simulink model "adc_to_10gbe"  (Simulink 7.4)
settings: Solver=ode45  StartTime=0.0  StopTime=200000  RelTol=1e-3
undefined symbols (not defined in the file): ROACH
libraries: xbsIndex_r4 x112, xps_library x77, casper_library_misc x6, xbsReplacements_r4 x3
(part 2 of 2)

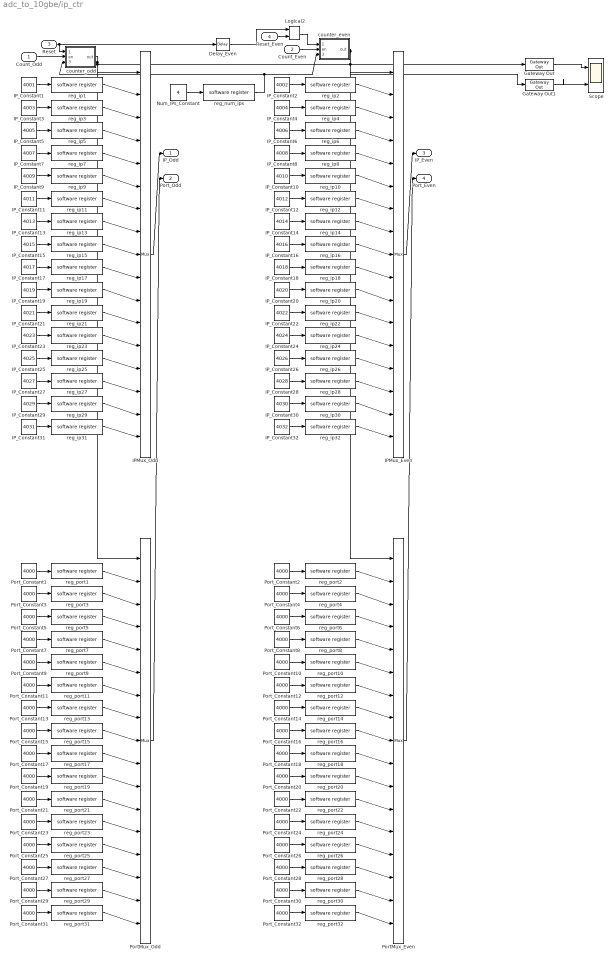
== system adc_to_10gbe/ip_ctr ==
  Count_Odd : Inport  OutDataType=sfix(16)  OutScaling=2^0
  Count_Even : Inport  Port=2  OutDataType=sfix(16)  OutScaling=2^0
  Reset : Inport  Port=3  OutDataType=sfix(16)  OutScaling=2^0
  Reset_Even : Inport  Port=4  OutDataType=sfix(16)  OutScaling=2^0
  Delay_Even : xbsIndex_r4/Delay  en=off  latency=4  dbl_ovrd=off  reg_retiming=off  block_type=delay
      settings: xl_area=[0, 0, 0, 0, 0, 0, 0]  block_version=10.1
  Gateway Out : xbsIndex_r4/Gateway Out  hdl_port=on  timing_constraint=None  locs_specified=off  LOCs={}  block_type=gatewayout
      settings: infoedit="Gateway out block.  Converts Xilinx fixed point inputs into ouputs of type Simulink integer, double, or fixed point.<P><P>Hardware notes:  In hardware these blocks become top level output ports or are discarded, depending on how they are configured."  xl_area=[0, 0, 0, 0, 0, 0, 0]  block_version=10.1
  Gateway Out1 : xbsIndex_r4/Gateway Out  hdl_port=on  timing_constraint=None  locs_specified=off  LOCs={}  block_type=gatewayout
      settings: infoedit="Gateway out block.  Converts Xilinx fixed point inputs into ouputs of type Simulink integer, double, or fixed point.<P><P>Hardware notes:  In hardware these blocks become top level output ports or are discarded, depending on how they are configured."  xl_area=[0, 0, 0, 0, 0, 0, 0]  block_version=10.1
  IPMux_Even : xbsIndex_r4/Mux  inputs=16  en=off  latency=3  precision=Full  arith_type="Signed  (2's comp)"  n_bits=8  bin_pt=2  quantization=Truncate  overflow=Wrap  dbl_ovrd=off  block_type=mux
      settings: xl_area=[0, 0, 0, 0, 0, 0, 0]  block_version=10.1
  IPMux_Odd : xbsIndex_r4/Mux  inputs=16  en=off  latency=3  precision=Full  arith_type="Signed  (2's comp)"  n_bits=8  bin_pt=2  quantization=Truncate  overflow=Wrap  dbl_ovrd=off  block_type=mux
      settings: xl_area=[0, 0, 0, 0, 0, 0, 0]  block_version=10.1
  IP_Constant1 : Constant  Value=4001  OutDataType=sfix(16)  OutScaling=2^0
  IP_Constant10 : Constant  Value=4010  OutDataType=sfix(16)  OutScaling=2^0
  IP_Constant11 : Constant  Value=4011  OutDataType=sfix(16)  OutScaling=2^0
  IP_Constant12 : Constant  Value=4012  OutDataType=sfix(16)  OutScaling=2^0
  IP_Constant13 : Constant  Value=4013  OutDataType=sfix(16)  OutScaling=2^0
  IP_Constant14 : Constant  Value=4014  OutDataType=sfix(16)  OutScaling=2^0
  IP_Constant15 : Constant  Value=4015  OutDataType=sfix(16)  OutScaling=2^0
  IP_Constant16 : Constant  Value=4016  OutDataType=sfix(16)  OutScaling=2^0
  IP_Constant17 : Constant  Value=4017  OutDataType=sfix(16)  OutScaling=2^0
  IP_Constant18 : Constant  Value=4018  OutDataType=sfix(16)  OutScaling=2^0
  IP_Constant19 : Constant  Value=4019  OutDataType=sfix(16)  OutScaling=2^0
  IP_Constant2 : Constant  Value=4002  OutDataType=sfix(16)  OutScaling=2^0
  IP_Constant20 : Constant  Value=4020  OutDataType=sfix(16)  OutScaling=2^0
  IP_Constant21 : Constant  Value=4021  OutDataType=sfix(16)  OutScaling=2^0
  IP_Constant22 : Constant  Value=4022  OutDataType=sfix(16)  OutScaling=2^0
  IP_Constant23 : Constant  Value=4023  OutDataType=sfix(16)  OutScaling=2^0
  IP_Constant24 : Constant  Value=4024  OutDataType=sfix(16)  OutScaling=2^0
  IP_Constant25 : Constant  Value=4025  OutDataType=sfix(16)  OutScaling=2^0
  IP_Constant26 : Constant  Value=4026  OutDataType=sfix(16)  OutScaling=2^0
  IP_Constant27 : Constant  Value=4027  OutDataType=sfix(16)  OutScaling=2^0
  IP_Constant28 : Constant  Value=4028  OutDataType=sfix(16)  OutScaling=2^0
  IP_Constant29 : Constant  Value=4029  OutDataType=sfix(16)  OutScaling=2^0
  IP_Constant3 : Constant  Value=4003  OutDataType=sfix(16)  OutScaling=2^0
  IP_Constant30 : Constant  Value=4030  OutDataType=sfix(16)  OutScaling=2^0
  IP_Constant31 : Constant  Value=4031  OutDataType=sfix(16)  OutScaling=2^0
  IP_Constant32 : Constant  Value=4032  OutDataType=sfix(16)  OutScaling=2^0
  IP_Constant4 : Constant  Value=4004  OutDataType=sfix(16)  OutScaling=2^0
  IP_Constant5 : Constant  Value=4005  OutDataType=sfix(16)  OutScaling=2^0
  IP_Constant6 : Constant  Value=4006  OutDataType=sfix(16)  OutScaling=2^0
  IP_Constant7 : Constant  Value=4007  OutDataType=sfix(16)  OutScaling=2^0
  IP_Constant8 : Constant  Value=4008  OutDataType=sfix(16)  OutScaling=2^0
  IP_Constant9 : Constant  Value=4009  OutDataType=sfix(16)  OutScaling=2^0
  Logical2 : xbsIndex_r4/Logical  logical_function=OR  inputs=2  en=off  latency=0  precision=Full  arith_type=Unsigned  n_bits=8  bin_pt=2  align_bp=on  dbl_ovrd=off  block_type=logical
      settings: xl_area=[0, 0, 0, 0, 0, 0, 0]  block_version=10.1
  Num_IPs_Constant : Constant  Value=4  OutDataType=sfix(16)  OutScaling=2^0
  PortMux_Even : xbsIndex_r4/Mux  inputs=16  en=off  latency=3  precision=Full  arith_type="Signed  (2's comp)"  n_bits=8  bin_pt=2  quantization=Truncate  overflow=Wrap  dbl_ovrd=off  block_type=mux
      settings: xl_area=[0, 0, 0, 0, 0, 0, 0]  block_version=10.1
  PortMux_Odd : xbsIndex_r4/Mux  inputs=16  en=off  latency=3  precision=Full  arith_type="Signed  (2's comp)"  n_bits=8  bin_pt=2  quantization=Truncate  overflow=Wrap  dbl_ovrd=off  block_type=mux
      settings: xl_area=[0, 0, 0, 0, 0, 0, 0]  block_version=10.1
  Port_Constant{1..32} (32 alike) : Constant  Value=4000  OutDataType=sfix(16)  OutScaling=2^0
  Scope : Scope  NumInputPorts=2
      settings: YMin=-5~-5  YMax=5~5  SaveName=ScopeData4
  counter_even : Subsystem
  counter_odd : Subsystem
  reg_ip1 : xps_library/software register  Tag=xps:sw_reg  SystemSampleTime=-1  io_dir=From Processor  arith_type=Unsigned  bitwidth=32  bin_pt=0  sample_period=1  gw_name=adc_to_10gbe_ip_ctr_reg_ip1_user_data_out
      link override adc_to_10gbe_ip_ctr_reg_ip1_user_data_out: arith_type=Unsigned  n_bits=32  bin_pt=0  period=1
      link override adc_to_10gbe_mod_ip_ctr_reg_ip1_user_data_out: arith_type=Unsigned  n_bits=32  bin_pt=0  period=1
  reg_ip10 : xps_library/software register  Tag=xps:sw_reg  SystemSampleTime=-1  io_dir=From Processor  arith_type=Unsigned  bitwidth=32  bin_pt=0  sample_period=1  gw_name=adc_to_10gbe_ip_ctr_reg_ip10_user_data_out
      link override adc_to_10gbe_ip_ctr_reg_ip10_user_data_out: arith_type=Unsigned  n_bits=32  bin_pt=0  period=1
      link override adc_to_10gbe_mod_ip_ctr_reg_ip10_user_data_out: arith_type=Unsigned  n_bits=32  bin_pt=0  period=1
  reg_ip11 : xps_library/software register  Tag=xps:sw_reg  SystemSampleTime=-1  io_dir=From Processor  arith_type=Unsigned  bitwidth=32  bin_pt=0  sample_period=1  gw_name=adc_to_10gbe_ip_ctr_reg_ip11_user_data_out
      link override adc_to_10gbe_ip_ctr_reg_ip11_user_data_out: arith_type=Unsigned  n_bits=32  bin_pt=0  period=1
      link override adc_to_10gbe_mod_ip_ctr_reg_ip11_user_data_out: arith_type=Unsigned  n_bits=32  bin_pt=0  period=1
  reg_ip12 : xps_library/software register  Tag=xps:sw_reg  SystemSampleTime=-1  io_dir=From Processor  arith_type=Unsigned  bitwidth=32  bin_pt=0  sample_period=1  gw_name=adc_to_10gbe_ip_ctr_reg_ip12_user_data_out
      link override adc_to_10gbe_ip_ctr_reg_ip12_user_data_out: arith_type=Unsigned  n_bits=32  bin_pt=0  period=1
      link override adc_to_10gbe_mod_ip_ctr_reg_ip12_user_data_out: arith_type=Unsigned  n_bits=32  bin_pt=0  period=1
  reg_ip13 : xps_library/software register  Tag=xps:sw_reg  SystemSampleTime=-1  io_dir=From Processor  arith_type=Unsigned  bitwidth=32  bin_pt=0  sample_period=1  gw_name=adc_to_10gbe_ip_ctr_reg_ip13_user_data_out
      link override adc_to_10gbe_ip_ctr_reg_ip13_user_data_out: arith_type=Unsigned  n_bits=32  bin_pt=0  period=1
      link override adc_to_10gbe_mod_ip_ctr_reg_ip13_user_data_out: arith_type=Unsigned  n_bits=32  bin_pt=0  period=1
  reg_ip14 : xps_library/software register  Tag=xps:sw_reg  SystemSampleTime=-1  io_dir=From Processor  arith_type=Unsigned  bitwidth=32  bin_pt=0  sample_period=1  gw_name=adc_to_10gbe_ip_ctr_reg_ip14_user_data_out
      link override adc_to_10gbe_ip_ctr_reg_ip14_user_data_out: arith_type=Unsigned  n_bits=32  bin_pt=0  period=1
      link override adc_to_10gbe_mod_ip_ctr_reg_ip14_user_data_out: arith_type=Unsigned  n_bits=32  bin_pt=0  period=1
  reg_ip15 : xps_library/software register  Tag=xps:sw_reg  SystemSampleTime=-1  io_dir=From Processor  arith_type=Unsigned  bitwidth=32  bin_pt=0  sample_period=1  gw_name=adc_to_10gbe_ip_ctr_reg_ip15_user_data_out
      link override adc_to_10gbe_ip_ctr_reg_ip15_user_data_out: arith_type=Unsigned  n_bits=32  bin_pt=0  period=1
      link override adc_to_10gbe_mod_ip_ctr_reg_ip15_user_data_out: arith_type=Unsigned  n_bits=32  bin_pt=0  period=1
  reg_ip16 : xps_library/software register  Tag=xps:sw_reg  SystemSampleTime=-1  io_dir=From Processor  arith_type=Unsigned  bitwidth=32  bin_pt=0  sample_period=1  gw_name=adc_to_10gbe_ip_ctr_reg_ip16_user_data_out
      link override adc_to_10gbe_ip_ctr_reg_ip16_user_data_out: arith_type=Unsigned  n_bits=32  bin_pt=0  period=1
      link override adc_to_10gbe_mod_ip_ctr_reg_ip16_user_data_out: arith_type=Unsigned  n_bits=32  bin_pt=0  period=1
  reg_ip17 : xps_library/software register  Tag=xps:sw_reg  SystemSampleTime=-1  io_dir=From Processor  arith_type=Unsigned  bitwidth=32  bin_pt=0  sample_period=1  gw_name=adc_to_10gbe_ip_ctr_reg_ip17_user_data_out
      link override adc_to_10gbe_ip_ctr_reg_ip17_user_data_out: arith_type=Unsigned  n_bits=32  bin_pt=0  period=1
      link override adc_to_10gbe_mod_ip_ctr_reg_ip17_user_data_out: arith_type=Unsigned  n_bits=32  bin_pt=0  period=1
  reg_ip18 : xps_library/software register  Tag=xps:sw_reg  SystemSampleTime=-1  io_dir=From Processor  arith_type=Unsigned  bitwidth=32  bin_pt=0  sample_period=1  gw_name=adc_to_10gbe_ip_ctr_reg_ip18_user_data_out
      link override adc_to_10gbe_ip_ctr_reg_ip18_user_data_out: arith_type=Unsigned  n_bits=32  bin_pt=0  period=1
      link override adc_to_10gbe_mod_ip_ctr_reg_ip18_user_data_out: arith_type=Unsigned  n_bits=32  bin_pt=0  period=1
  reg_ip19 : xps_library/software register  Tag=xps:sw_reg  SystemSampleTime=-1  io_dir=From Processor  arith_type=Unsigned  bitwidth=32  bin_pt=0  sample_period=1  gw_name=adc_to_10gbe_ip_ctr_reg_ip19_user_data_out
      link override adc_to_10gbe_ip_ctr_reg_ip19_user_data_out: arith_type=Unsigned  n_bits=32  bin_pt=0  period=1
      link override adc_to_10gbe_mod_ip_ctr_reg_ip19_user_data_out: arith_type=Unsigned  n_bits=32  bin_pt=0  period=1
  reg_ip2 : xps_library/software register  Tag=xps:sw_reg  SystemSampleTime=-1  io_dir=From Processor  arith_type=Unsigned  bitwidth=32  bin_pt=0  sample_period=1  gw_name=adc_to_10gbe_ip_ctr_reg_ip2_user_data_out
      link override adc_to_10gbe_ip_ctr_reg_ip2_user_data_out: arith_type=Unsigned  n_bits=32  bin_pt=0  period=1
      link override adc_to_10gbe_mod_ip_ctr_reg_ip2_user_data_out: arith_type=Unsigned  n_bits=32  bin_pt=0  period=1
  reg_ip20 : xps_library/software register  Tag=xps:sw_reg  SystemSampleTime=-1  io_dir=From Processor  arith_type=Unsigned  bitwidth=32  bin_pt=0  sample_period=1  gw_name=adc_to_10gbe_ip_ctr_reg_ip20_user_data_out
      link override adc_to_10gbe_ip_ctr_reg_ip20_user_data_out: arith_type=Unsigned  n_bits=32  bin_pt=0  period=1
      link override adc_to_10gbe_mod_ip_ctr_reg_ip20_user_data_out: arith_type=Unsigned  n_bits=32  bin_pt=0  period=1
  reg_ip21 : xps_library/software register  Tag=xps:sw_reg  SystemSampleTime=-1  io_dir=From Processor  arith_type=Unsigned  bitwidth=32  bin_pt=0  sample_period=1  gw_name=adc_to_10gbe_ip_ctr_reg_ip21_user_data_out
      link override adc_to_10gbe_ip_ctr_reg_ip21_user_data_out: arith_type=Unsigned  n_bits=32  bin_pt=0  period=1
      link override adc_to_10gbe_mod_ip_ctr_reg_ip21_user_data_out: arith_type=Unsigned  n_bits=32  bin_pt=0  period=1
  reg_ip22 : xps_library/software register  Tag=xps:sw_reg  SystemSampleTime=-1  io_dir=From Processor  arith_type=Unsigned  bitwidth=32  bin_pt=0  sample_period=1  gw_name=adc_to_10gbe_ip_ctr_reg_ip22_user_data_out
      link override adc_to_10gbe_ip_ctr_reg_ip22_user_data_out: arith_type=Unsigned  n_bits=32  bin_pt=0  period=1
      link override adc_to_10gbe_mod_ip_ctr_reg_ip22_user_data_out: arith_type=Unsigned  n_bits=32  bin_pt=0  period=1
  reg_ip23 : xps_library/software register  Tag=xps:sw_reg  SystemSampleTime=-1  io_dir=From Processor  arith_type=Unsigned  bitwidth=32  bin_pt=0  sample_period=1  gw_name=adc_to_10gbe_ip_ctr_reg_ip23_user_data_out
      link override adc_to_10gbe_ip_ctr_reg_ip23_user_data_out: arith_type=Unsigned  n_bits=32  bin_pt=0  period=1
      link override adc_to_10gbe_mod_ip_ctr_reg_ip23_user_data_out: arith_type=Unsigned  n_bits=32  bin_pt=0  period=1
  reg_ip24 : xps_library/software register  Tag=xps:sw_reg  SystemSampleTime=-1  io_dir=From Processor  arith_type=Unsigned  bitwidth=32  bin_pt=0  sample_period=1  gw_name=adc_to_10gbe_ip_ctr_reg_ip24_user_data_out
      link override adc_to_10gbe_ip_ctr_reg_ip24_user_data_out: arith_type=Unsigned  n_bits=32  bin_pt=0  period=1
      link override adc_to_10gbe_mod_ip_ctr_reg_ip24_user_data_out: arith_type=Unsigned  n_bits=32  bin_pt=0  period=1
  reg_ip25 : xps_library/software register  Tag=xps:sw_reg  SystemSampleTime=-1  io_dir=From Processor  arith_type=Unsigned  bitwidth=32  bin_pt=0  sample_period=1  gw_name=adc_to_10gbe_ip_ctr_reg_ip25_user_data_out
      link override adc_to_10gbe_ip_ctr_reg_ip25_user_data_out: arith_type=Unsigned  n_bits=32  bin_pt=0  period=1
      link override adc_to_10gbe_mod_ip_ctr_reg_ip25_user_data_out: arith_type=Unsigned  n_bits=32  bin_pt=0  period=1
  reg_ip26 : xps_library/software register  Tag=xps:sw_reg  SystemSampleTime=-1  io_dir=From Processor  arith_type=Unsigned  bitwidth=32  bin_pt=0  sample_period=1  gw_name=adc_to_10gbe_ip_ctr_reg_ip26_user_data_out
      link override adc_to_10gbe_ip_ctr_reg_ip26_user_data_out: arith_type=Unsigned  n_bits=32  bin_pt=0  period=1
      link override adc_to_10gbe_mod_ip_ctr_reg_ip26_user_data_out: arith_type=Unsigned  n_bits=32  bin_pt=0  period=1
  reg_ip27 : xps_library/software register  Tag=xps:sw_reg  SystemSampleTime=-1  io_dir=From Processor  arith_type=Unsigned  bitwidth=32  bin_pt=0  sample_period=1  gw_name=adc_to_10gbe_ip_ctr_reg_ip27_user_data_out
      link override adc_to_10gbe_ip_ctr_reg_ip27_user_data_out: arith_type=Unsigned  n_bits=32  bin_pt=0  period=1
      link override adc_to_10gbe_mod_ip_ctr_reg_ip27_user_data_out: arith_type=Unsigned  n_bits=32  bin_pt=0  period=1
  reg_ip28 : xps_library/software register  Tag=xps:sw_reg  SystemSampleTime=-1  io_dir=From Processor  arith_type=Unsigned  bitwidth=32  bin_pt=0  sample_period=1  gw_name=adc_to_10gbe_ip_ctr_reg_ip28_user_data_out
      link override adc_to_10gbe_ip_ctr_reg_ip28_user_data_out: arith_type=Unsigned  n_bits=32  bin_pt=0  period=1
      link override adc_to_10gbe_mod_ip_ctr_reg_ip28_user_data_out: arith_type=Unsigned  n_bits=32  bin_pt=0  period=1
  reg_ip29 : xps_library/software register  Tag=xps:sw_reg  SystemSampleTime=-1  io_dir=From Processor  arith_type=Unsigned  bitwidth=32  bin_pt=0  sample_period=1  gw_name=adc_to_10gbe_ip_ctr_reg_ip29_user_data_out
      link override adc_to_10gbe_ip_ctr_reg_ip29_user_data_out: arith_type=Unsigned  n_bits=32  bin_pt=0  period=1
      link override adc_to_10gbe_mod_ip_ctr_reg_ip29_user_data_out: arith_type=Unsigned  n_bits=32  bin_pt=0  period=1
  reg_ip3 : xps_library/software register  Tag=xps:sw_reg  SystemSampleTime=-1  io_dir=From Processor  arith_type=Unsigned  bitwidth=32  bin_pt=0  sample_period=1  gw_name=adc_to_10gbe_ip_ctr_reg_ip3_user_data_out
      link override adc_to_10gbe_ip_ctr_reg_ip3_user_data_out: arith_type=Unsigned  n_bits=32  bin_pt=0  period=1
      link override adc_to_10gbe_mod_ip_ctr_reg_ip3_user_data_out: arith_type=Unsigned  n_bits=32  bin_pt=0  period=1
  reg_ip30 : xps_library/software register  Tag=xps:sw_reg  SystemSampleTime=-1  io_dir=From Processor  arith_type=Unsigned  bitwidth=32  bin_pt=0  sample_period=1  gw_name=adc_to_10gbe_ip_ctr_reg_ip30_user_data_out
      link override adc_to_10gbe_ip_ctr_reg_ip30_user_data_out: arith_type=Unsigned  n_bits=32  bin_pt=0  period=1
      link override adc_to_10gbe_mod_ip_ctr_reg_ip30_user_data_out: arith_type=Unsigned  n_bits=32  bin_pt=0  period=1
  reg_ip31 : xps_library/software register  Tag=xps:sw_reg  SystemSampleTime=-1  io_dir=From Processor  arith_type=Unsigned  bitwidth=32  bin_pt=0  sample_period=1  gw_name=adc_to_10gbe_ip_ctr_reg_ip31_user_data_out
      link override adc_to_10gbe_ip_ctr_reg_ip31_user_data_out: arith_type=Unsigned  n_bits=32  bin_pt=0  period=1
      link override adc_to_10gbe_mod_ip_ctr_reg_ip31_user_data_out: arith_type=Unsigned  n_bits=32  bin_pt=0  period=1
  reg_ip32 : xps_library/software register  Tag=xps:sw_reg  SystemSampleTime=-1  io_dir=From Processor  arith_type=Unsigned  bitwidth=32  bin_pt=0  sample_period=1  gw_name=adc_to_10gbe_ip_ctr_reg_ip32_user_data_out
      link override adc_to_10gbe_ip_ctr_reg_ip32_user_data_out: arith_type=Unsigned  n_bits=32  bin_pt=0  period=1
      link override adc_to_10gbe_mod_ip_ctr_reg_ip32_user_data_out: arith_type=Unsigned  n_bits=32  bin_pt=0  period=1
  reg_ip4 : xps_library/software register  Tag=xps:sw_reg  SystemSampleTime=-1  io_dir=From Processor  arith_type=Unsigned  bitwidth=32  bin_pt=0  sample_period=1  gw_name=adc_to_10gbe_ip_ctr_reg_ip4_user_data_out
      link override adc_to_10gbe_ip_ctr_reg_ip4_user_data_out: arith_type=Unsigned  n_bits=32  bin_pt=0  period=1
      link override adc_to_10gbe_mod_ip_ctr_reg_ip4_user_data_out: arith_type=Unsigned  n_bits=32  bin_pt=0  period=1
  reg_ip5 : xps_library/software register  Tag=xps:sw_reg  SystemSampleTime=-1  io_dir=From Processor  arith_type=Unsigned  bitwidth=32  bin_pt=0  sample_period=1  gw_name=adc_to_10gbe_ip_ctr_reg_ip5_user_data_out
      link override adc_to_10gbe_ip_ctr_reg_ip5_user_data_out: arith_type=Unsigned  n_bits=32  bin_pt=0  period=1
      link override adc_to_10gbe_mod_ip_ctr_reg_ip5_user_data_out: arith_type=Unsigned  n_bits=32  bin_pt=0  period=1
  reg_ip6 : xps_library/software register  Tag=xps:sw_reg  SystemSampleTime=-1  io_dir=From Processor  arith_type=Unsigned  bitwidth=32  bin_pt=0  sample_period=1  gw_name=adc_to_10gbe_ip_ctr_reg_ip6_user_data_out
      link override adc_to_10gbe_ip_ctr_reg_ip6_user_data_out: arith_type=Unsigned  n_bits=32  bin_pt=0  period=1
      link override adc_to_10gbe_mod_ip_ctr_reg_ip6_user_data_out: arith_type=Unsigned  n_bits=32  bin_pt=0  period=1
  reg_ip7 : xps_library/software register  Tag=xps:sw_reg  SystemSampleTime=-1  io_dir=From Processor  arith_type=Unsigned  bitwidth=32  bin_pt=0  sample_period=1  gw_name=adc_to_10gbe_ip_ctr_reg_ip7_user_data_out
      link override adc_to_10gbe_ip_ctr_reg_ip7_user_data_out: arith_type=Unsigned  n_bits=32  bin_pt=0  period=1
      link override adc_to_10gbe_mod_ip_ctr_reg_ip7_user_data_out: arith_type=Unsigned  n_bits=32  bin_pt=0  period=1
  reg_ip8 : xps_library/software register  Tag=xps:sw_reg  SystemSampleTime=-1  io_dir=From Processor  arith_type=Unsigned  bitwidth=32  bin_pt=0  sample_period=1  gw_name=adc_to_10gbe_ip_ctr_reg_ip8_user_data_out
      link override adc_to_10gbe_ip_ctr_reg_ip8_user_data_out: arith_type=Unsigned  n_bits=32  bin_pt=0  period=1
      link override adc_to_10gbe_mod_ip_ctr_reg_ip8_user_data_out: arith_type=Unsigned  n_bits=32  bin_pt=0  period=1
  reg_ip9 : xps_library/software register  Tag=xps:sw_reg  SystemSampleTime=-1  io_dir=From Processor  arith_type=Unsigned  bitwidth=32  bin_pt=0  sample_period=1  gw_name=adc_to_10gbe_ip_ctr_reg_ip9_user_data_out
      link override adc_to_10gbe_ip_ctr_reg_ip9_user_data_out: arith_type=Unsigned  n_bits=32  bin_pt=0  period=1
      link override adc_to_10gbe_mod_ip_ctr_reg_ip9_user_data_out: arith_type=Unsigned  n_bits=32  bin_pt=0  period=1
  reg_num_ips : xps_library/software register  Tag=xps:sw_reg  SystemSampleTime=-1  io_dir=From Processor  arith_type=Unsigned  bitwidth=32  bin_pt=0  sample_period=1  gw_name=adc_to_10gbe_ip_ctr_reg_num_ips_user_data_out
      link override adc_to_10gbe_ip_ctr_reg_num_ips_user_data_out: arith_type=Unsigned  n_bits=32  bin_pt=0  period=1
      link override adc_to_10gbe_mod_ip_ctr_reg_num_ips_user_data_out: arith_type=Unsigned  n_bits=32  bin_pt=0  period=1
  reg_port1 : xps_library/software register  Tag=xps:sw_reg  SystemSampleTime=-1  io_dir=From Processor  arith_type=Unsigned  bitwidth=32  bin_pt=0  sample_period=1  gw_name=adc_to_10gbe_ip_ctr_reg_port1_user_data_out
      link override adc_to_10gbe_ip_ctr_reg_port1_user_data_out: arith_type=Unsigned  n_bits=32  bin_pt=0  period=1
      link override adc_to_10gbe_mod_ip_ctr_reg_port1_user_data_out: arith_type=Unsigned  n_bits=32  bin_pt=0  period=1
  reg_port10 : xps_library/software register  Tag=xps:sw_reg  SystemSampleTime=-1  io_dir=From Processor  arith_type=Unsigned  bitwidth=32  bin_pt=0  sample_period=1  gw_name=adc_to_10gbe_ip_ctr_reg_port10_user_data_out
      link override adc_to_10gbe_ip_ctr_reg_port10_user_data_out: arith_type=Unsigned  n_bits=32  bin_pt=0  period=1
      link override adc_to_10gbe_mod_ip_ctr_reg_port10_user_data_out: arith_type=Unsigned  n_bits=32  bin_pt=0  period=1
  reg_port11 : xps_library/software register  Tag=xps:sw_reg  SystemSampleTime=-1  io_dir=From Processor  arith_type=Unsigned  bitwidth=32  bin_pt=0  sample_period=1  gw_name=adc_to_10gbe_ip_ctr_reg_port11_user_data_out
      link override adc_to_10gbe_ip_ctr_reg_port11_user_data_out: arith_type=Unsigned  n_bits=32  bin_pt=0  period=1
      link override adc_to_10gbe_mod_ip_ctr_reg_port11_user_data_out: arith_type=Unsigned  n_bits=32  bin_pt=0  period=1
  reg_port12 : xps_library/software register  Tag=xps:sw_reg  SystemSampleTime=-1  io_dir=From Processor  arith_type=Unsigned  bitwidth=32  bin_pt=0  sample_period=1  gw_name=adc_to_10gbe_ip_ctr_reg_port12_user_data_out
      link override adc_to_10gbe_ip_ctr_reg_port12_user_data_out: arith_type=Unsigned  n_bits=32  bin_pt=0  period=1
      link override adc_to_10gbe_mod_ip_ctr_reg_port12_user_data_out: arith_type=Unsigned  n_bits=32  bin_pt=0  period=1
  reg_port13 : xps_library/software register  Tag=xps:sw_reg  SystemSampleTime=-1  io_dir=From Processor  arith_type=Unsigned  bitwidth=32  bin_pt=0  sample_period=1  gw_name=adc_to_10gbe_ip_ctr_reg_port13_user_data_out
      link override adc_to_10gbe_ip_ctr_reg_port13_user_data_out: arith_type=Unsigned  n_bits=32  bin_pt=0  period=1
      link override adc_to_10gbe_mod_ip_ctr_reg_port13_user_data_out: arith_type=Unsigned  n_bits=32  bin_pt=0  period=1
  reg_port14 : xps_library/software register  Tag=xps:sw_reg  SystemSampleTime=-1  io_dir=From Processor  arith_type=Unsigned  bitwidth=32  bin_pt=0  sample_period=1  gw_name=adc_to_10gbe_ip_ctr_reg_port14_user_data_out
      link override adc_to_10gbe_ip_ctr_reg_port14_user_data_out: arith_type=Unsigned  n_bits=32  bin_pt=0  period=1
      link override adc_to_10gbe_mod_ip_ctr_reg_port14_user_data_out: arith_type=Unsigned  n_bits=32  bin_pt=0  period=1
  reg_port15 : xps_library/software register  Tag=xps:sw_reg  SystemSampleTime=-1  io_dir=From Processor  arith_type=Unsigned  bitwidth=32  bin_pt=0  sample_period=1  gw_name=adc_to_10gbe_ip_ctr_reg_port15_user_data_out
      link override adc_to_10gbe_ip_ctr_reg_port15_user_data_out: arith_type=Unsigned  n_bits=32  bin_pt=0  period=1
      link override adc_to_10gbe_mod_ip_ctr_reg_port15_user_data_out: arith_type=Unsigned  n_bits=32  bin_pt=0  period=1
  reg_port16 : xps_library/software register  Tag=xps:sw_reg  SystemSampleTime=-1  io_dir=From Processor  arith_type=Unsigned  bitwidth=32  bin_pt=0  sample_period=1  gw_name=adc_to_10gbe_ip_ctr_reg_port16_user_data_out
      link override adc_to_10gbe_ip_ctr_reg_port16_user_data_out: arith_type=Unsigned  n_bits=32  bin_pt=0  period=1
      link override adc_to_10gbe_mod_ip_ctr_reg_port16_user_data_out: arith_type=Unsigned  n_bits=32  bin_pt=0  period=1
  reg_port17 : xps_library/software register  Tag=xps:sw_reg  SystemSampleTime=-1  io_dir=From Processor  arith_type=Unsigned  bitwidth=32  bin_pt=0  sample_period=1  gw_name=adc_to_10gbe_ip_ctr_reg_port17_user_data_out
      link override adc_to_10gbe_ip_ctr_reg_port17_user_data_out: arith_type=Unsigned  n_bits=32  bin_pt=0  period=1
      link override adc_to_10gbe_mod_ip_ctr_reg_port17_user_data_out: arith_type=Unsigned  n_bits=32  bin_pt=0  period=1
  reg_port18 : xps_library/software register  Tag=xps:sw_reg  SystemSampleTime=-1  io_dir=From Processor  arith_type=Unsigned  bitwidth=32  bin_pt=0  sample_period=1  gw_name=adc_to_10gbe_ip_ctr_reg_port18_user_data_out
      link override adc_to_10gbe_ip_ctr_reg_port18_user_data_out: arith_type=Unsigned  n_bits=32  bin_pt=0  period=1
      link override adc_to_10gbe_mod_ip_ctr_reg_port18_user_data_out: arith_type=Unsigned  n_bits=32  bin_pt=0  period=1
  reg_port19 : xps_library/software register  Tag=xps:sw_reg  SystemSampleTime=-1  io_dir=From Processor  arith_type=Unsigned  bitwidth=32  bin_pt=0  sample_period=1  gw_name=adc_to_10gbe_ip_ctr_reg_port19_user_data_out
      link override adc_to_10gbe_ip_ctr_reg_port19_user_data_out: arith_type=Unsigned  n_bits=32  bin_pt=0  period=1
      link override adc_to_10gbe_mod_ip_ctr_reg_port19_user_data_out: arith_type=Unsigned  n_bits=32  bin_pt=0  period=1
  reg_port2 : xps_library/software register  Tag=xps:sw_reg  SystemSampleTime=-1  io_dir=From Processor  arith_type=Unsigned  bitwidth=32  bin_pt=0  sample_period=1  gw_name=adc_to_10gbe_ip_ctr_reg_port2_user_data_out
      link override adc_to_10gbe_ip_ctr_reg_port2_user_data_out: arith_type=Unsigned  n_bits=32  bin_pt=0  period=1
      link override adc_to_10gbe_mod_ip_ctr_reg_port2_user_data_out: arith_type=Unsigned  n_bits=32  bin_pt=0  period=1
  reg_port20 : xps_library/software register  Tag=xps:sw_reg  SystemSampleTime=-1  io_dir=From Processor  arith_type=Unsigned  bitwidth=32  bin_pt=0  sample_period=1  gw_name=adc_to_10gbe_ip_ctr_reg_port20_user_data_out
      link override adc_to_10gbe_ip_ctr_reg_port20_user_data_out: arith_type=Unsigned  n_bits=32  bin_pt=0  period=1
      link override adc_to_10gbe_mod_ip_ctr_reg_port20_user_data_out: arith_type=Unsigned  n_bits=32  bin_pt=0  period=1
  reg_port21 : xps_library/software register  Tag=xps:sw_reg  SystemSampleTime=-1  io_dir=From Processor  arith_type=Unsigned  bitwidth=32  bin_pt=0  sample_period=1  gw_name=adc_to_10gbe_ip_ctr_reg_port21_user_data_out
      link override adc_to_10gbe_ip_ctr_reg_port21_user_data_out: arith_type=Unsigned  n_bits=32  bin_pt=0  period=1
      link override adc_to_10gbe_mod_ip_ctr_reg_port21_user_data_out: arith_type=Unsigned  n_bits=32  bin_pt=0  period=1
  reg_port22 : xps_library/software register  Tag=xps:sw_reg  SystemSampleTime=-1  io_dir=From Processor  arith_type=Unsigned  bitwidth=32  bin_pt=0  sample_period=1  gw_name=adc_to_10gbe_ip_ctr_reg_port22_user_data_out
      link override adc_to_10gbe_ip_ctr_reg_port22_user_data_out: arith_type=Unsigned  n_bits=32  bin_pt=0  period=1
      link override adc_to_10gbe_mod_ip_ctr_reg_port22_user_data_out: arith_type=Unsigned  n_bits=32  bin_pt=0  period=1
  reg_port23 : xps_library/software register  Tag=xps:sw_reg  SystemSampleTime=-1  io_dir=From Processor  arith_type=Unsigned  bitwidth=32  bin_pt=0  sample_period=1  gw_name=adc_to_10gbe_ip_ctr_reg_port23_user_data_out
      link override adc_to_10gbe_ip_ctr_reg_port23_user_data_out: arith_type=Unsigned  n_bits=32  bin_pt=0  period=1
      link override adc_to_10gbe_mod_ip_ctr_reg_port23_user_data_out: arith_type=Unsigned  n_bits=32  bin_pt=0  period=1
  reg_port24 : xps_library/software register  Tag=xps:sw_reg  SystemSampleTime=-1  io_dir=From Processor  arith_type=Unsigned  bitwidth=32  bin_pt=0  sample_period=1  gw_name=adc_to_10gbe_ip_ctr_reg_port24_user_data_out
      link override adc_to_10gbe_ip_ctr_reg_port24_user_data_out: arith_type=Unsigned  n_bits=32  bin_pt=0  period=1
      link override adc_to_10gbe_mod_ip_ctr_reg_port24_user_data_out: arith_type=Unsigned  n_bits=32  bin_pt=0  period=1
  reg_port25 : xps_library/software register  Tag=xps:sw_reg  SystemSampleTime=-1  io_dir=From Processor  arith_type=Unsigned  bitwidth=32  bin_pt=0  sample_period=1  gw_name=adc_to_10gbe_ip_ctr_reg_port25_user_data_out
      link override adc_to_10gbe_ip_ctr_reg_port25_user_data_out: arith_type=Unsigned  n_bits=32  bin_pt=0  period=1
      link override adc_to_10gbe_mod_ip_ctr_reg_port25_user_data_out: arith_type=Unsigned  n_bits=32  bin_pt=0  period=1
  reg_port26 : xps_library/software register  Tag=xps:sw_reg  SystemSampleTime=-1  io_dir=From Processor  arith_type=Unsigned  bitwidth=32  bin_pt=0  sample_period=1  gw_name=adc_to_10gbe_ip_ctr_reg_port26_user_data_out
      link override adc_to_10gbe_ip_ctr_reg_port26_user_data_out: arith_type=Unsigned  n_bits=32  bin_pt=0  period=1
      link override adc_to_10gbe_mod_ip_ctr_reg_port26_user_data_out: arith_type=Unsigned  n_bits=32  bin_pt=0  period=1
  reg_port27 : xps_library/software register  Tag=xps:sw_reg  SystemSampleTime=-1  io_dir=From Processor  arith_type=Unsigned  bitwidth=32  bin_pt=0  sample_period=1  gw_name=adc_to_10gbe_ip_ctr_reg_port27_user_data_out
      link override adc_to_10gbe_ip_ctr_reg_port27_user_data_out: arith_type=Unsigned  n_bits=32  bin_pt=0  period=1
      link override adc_to_10gbe_mod_ip_ctr_reg_port27_user_data_out: arith_type=Unsigned  n_bits=32  bin_pt=0  period=1
  reg_port28 : xps_library/software register  Tag=xps:sw_reg  SystemSampleTime=-1  io_dir=From Processor  arith_type=Unsigned  bitwidth=32  bin_pt=0  sample_period=1  gw_name=adc_to_10gbe_ip_ctr_reg_port28_user_data_out
      link override adc_to_10gbe_ip_ctr_reg_port28_user_data_out: arith_type=Unsigned  n_bits=32  bin_pt=0  period=1
      link override adc_to_10gbe_mod_ip_ctr_reg_port28_user_data_out: arith_type=Unsigned  n_bits=32  bin_pt=0  period=1
  reg_port29 : xps_library/software register  Tag=xps:sw_reg  SystemSampleTime=-1  io_dir=From Processor  arith_type=Unsigned  bitwidth=32  bin_pt=0  sample_period=1  gw_name=adc_to_10gbe_ip_ctr_reg_port29_user_data_out
      link override adc_to_10gbe_ip_ctr_reg_port29_user_data_out: arith_type=Unsigned  n_bits=32  bin_pt=0  period=1
      link override adc_to_10gbe_mod_ip_ctr_reg_port29_user_data_out: arith_type=Unsigned  n_bits=32  bin_pt=0  period=1
  reg_port3 : xps_library/software register  Tag=xps:sw_reg  SystemSampleTime=-1  io_dir=From Processor  arith_type=Unsigned  bitwidth=32  bin_pt=0  sample_period=1  gw_name=adc_to_10gbe_ip_ctr_reg_port3_user_data_out
      link override adc_to_10gbe_ip_ctr_reg_port3_user_data_out: arith_type=Unsigned  n_bits=32  bin_pt=0  period=1
      link override adc_to_10gbe_mod_ip_ctr_reg_port3_user_data_out: arith_type=Unsigned  n_bits=32  bin_pt=0  period=1
  reg_port30 : xps_library/software register  Tag=xps:sw_reg  SystemSampleTime=-1  io_dir=From Processor  arith_type=Unsigned  bitwidth=32  bin_pt=0  sample_period=1  gw_name=adc_to_10gbe_ip_ctr_reg_port30_user_data_out
      link override adc_to_10gbe_ip_ctr_reg_port30_user_data_out: arith_type=Unsigned  n_bits=32  bin_pt=0  period=1
      link override adc_to_10gbe_mod_ip_ctr_reg_port30_user_data_out: arith_type=Unsigned  n_bits=32  bin_pt=0  period=1
  reg_port31 : xps_library/software register  Tag=xps:sw_reg  SystemSampleTime=-1  io_dir=From Processor  arith_type=Unsigned  bitwidth=32  bin_pt=0  sample_period=1  gw_name=adc_to_10gbe_ip_ctr_reg_port31_user_data_out
      link override adc_to_10gbe_ip_ctr_reg_port31_user_data_out: arith_type=Unsigned  n_bits=32  bin_pt=0  period=1
      link override adc_to_10gbe_mod_ip_ctr_reg_port31_user_data_out: arith_type=Unsigned  n_bits=32  bin_pt=0  period=1
  reg_port32 : xps_library/software register  Tag=xps:sw_reg  SystemSampleTime=-1  io_dir=From Processor  arith_type=Unsigned  bitwidth=32  bin_pt=0  sample_period=1  gw_name=adc_to_10gbe_ip_ctr_reg_port32_user_data_out
      link override adc_to_10gbe_ip_ctr_reg_port32_user_data_out: arith_type=Unsigned  n_bits=32  bin_pt=0  period=1
      link override adc_to_10gbe_mod_ip_ctr_reg_port32_user_data_out: arith_type=Unsigned  n_bits=32  bin_pt=0  period=1
  reg_port4 : xps_library/software register  Tag=xps:sw_reg  SystemSampleTime=-1  io_dir=From Processor  arith_type=Unsigned  bitwidth=32  bin_pt=0  sample_period=1  gw_name=adc_to_10gbe_ip_ctr_reg_port4_user_data_out
      link override adc_to_10gbe_ip_ctr_reg_port4_user_data_out: arith_type=Unsigned  n_bits=32  bin_pt=0  period=1
      link override adc_to_10gbe_mod_ip_ctr_reg_port4_user_data_out: arith_type=Unsigned  n_bits=32  bin_pt=0  period=1
  reg_port5 : xps_library/software register  Tag=xps:sw_reg  SystemSampleTime=-1  io_dir=From Processor  arith_type=Unsigned  bitwidth=32  bin_pt=0  sample_period=1  gw_name=adc_to_10gbe_ip_ctr_reg_port5_user_data_out
      link override adc_to_10gbe_ip_ctr_reg_port5_user_data_out: arith_type=Unsigned  n_bits=32  bin_pt=0  period=1
      link override adc_to_10gbe_mod_ip_ctr_reg_port5_user_data_out: arith_type=Unsigned  n_bits=32  bin_pt=0  period=1
  reg_port6 : xps_library/software register  Tag=xps:sw_reg  SystemSampleTime=-1  io_dir=From Processor  arith_type=Unsigned  bitwidth=32  bin_pt=0  sample_period=1  gw_name=adc_to_10gbe_ip_ctr_reg_port6_user_data_out
      link override adc_to_10gbe_ip_ctr_reg_port6_user_data_out: arith_type=Unsigned  n_bits=32  bin_pt=0  period=1
      link override adc_to_10gbe_mod_ip_ctr_reg_port6_user_data_out: arith_type=Unsigned  n_bits=32  bin_pt=0  period=1
  reg_port7 : xps_library/software register  Tag=xps:sw_reg  SystemSampleTime=-1  io_dir=From Processor  arith_type=Unsigned  bitwidth=32  bin_pt=0  sample_period=1  gw_name=adc_to_10gbe_ip_ctr_reg_port7_user_data_out
      link override adc_to_10gbe_ip_ctr_reg_port7_user_data_out: arith_type=Unsigned  n_bits=32  bin_pt=0  period=1
      link override adc_to_10gbe_mod_ip_ctr_reg_port7_user_data_out: arith_type=Unsigned  n_bits=32  bin_pt=0  period=1
  reg_port8 : xps_library/software register  Tag=xps:sw_reg  SystemSampleTime=-1  io_dir=From Processor  arith_type=Unsigned  bitwidth=32  bin_pt=0  sample_period=1  gw_name=adc_to_10gbe_ip_ctr_reg_port8_user_data_out
      link override adc_to_10gbe_ip_ctr_reg_port8_user_data_out: arith_type=Unsigned  n_bits=32  bin_pt=0  period=1
      link override adc_to_10gbe_mod_ip_ctr_reg_port8_user_data_out: arith_type=Unsigned  n_bits=32  bin_pt=0  period=1
  reg_port9 : xps_library/software register  Tag=xps:sw_reg  SystemSampleTime=-1  io_dir=From Processor  arith_type=Unsigned  bitwidth=32  bin_pt=0  sample_period=1  gw_name=adc_to_10gbe_ip_ctr_reg_port9_user_data_out
      link override adc_to_10gbe_ip_ctr_reg_port9_user_data_out: arith_type=Unsigned  n_bits=32  bin_pt=0  period=1
      link override adc_to_10gbe_mod_ip_ctr_reg_port9_user_data_out: arith_type=Unsigned  n_bits=32  bin_pt=0  period=1
  IP_Odd : Outport  OutDataType=sfix(16)  OutScaling=2^0
  Port_Odd : Outport  Port=2  OutDataType=sfix(16)  OutScaling=2^0
  IP_Even : Outport  Port=3  OutDataType=sfix(16)  OutScaling=2^0
  Port_Even : Outport  Port=4  OutDataType=sfix(16)  OutScaling=2^0
  wires:
  Reset/1 -> Delay_Even/1, counter_odd/1(sync_in)
  Count_Odd/1 -> counter_odd/2(en)
  counter_odd/1(out) -> IPMux_Odd/1, PortMux_Odd/1, Gateway Out/1
  IPMux_Odd/1 -> IP_Odd/1
  PortMux_Odd/1 -> Port_Odd/1
  Count_Even/1 -> counter_even/2(en)
  counter_even/1(out) -> IPMux_Even/1, PortMux_Even/1, Gateway Out1/1
  IPMux_Even/1 -> IP_Even/1
  PortMux_Even/1 -> Port_Even/1
  IP_Constant1/1 -> reg_ip1/1
  reg_ip1/1 -> IPMux_Odd/2
  Port_Constant1/1 -> reg_port1/1
  reg_port1/1 -> PortMux_Odd/2
  IP_Constant3/1 -> reg_ip3/1
  reg_ip3/1 -> IPMux_Odd/3
  Port_Constant3/1 -> reg_port3/1
  reg_port3/1 -> PortMux_Odd/3
  IP_Constant5/1 -> reg_ip5/1
  reg_ip5/1 -> IPMux_Odd/4
  Port_Constant5/1 -> reg_port5/1
  reg_port5/1 -> PortMux_Odd/4
  IP_Constant7/1 -> reg_ip7/1
  reg_ip7/1 -> IPMux_Odd/5
  Port_Constant7/1 -> reg_port7/1
  reg_port7/1 -> PortMux_Odd/5
  IP_Constant9/1 -> reg_ip9/1
  reg_ip9/1 -> IPMux_Odd/6
  Port_Constant9/1 -> reg_port9/1
  reg_port9/1 -> PortMux_Odd/6
  IP_Constant11/1 -> reg_ip11/1
  reg_ip11/1 -> IPMux_Odd/7
  Port_Constant11/1 -> reg_port11/1
  reg_port11/1 -> PortMux_Odd/7
  IP_Constant13/1 -> reg_ip13/1
  reg_ip13/1 -> IPMux_Odd/8
  Port_Constant13/1 -> reg_port13/1
  reg_port13/1 -> PortMux_Odd/8
  IP_Constant15/1 -> reg_ip15/1
  reg_ip15/1 -> IPMux_Odd/9
  Port_Constant15/1 -> reg_port15/1
  reg_port15/1 -> PortMux_Odd/9
  IP_Constant17/1 -> reg_ip17/1
  reg_ip17/1 -> IPMux_Odd/10
  Port_Constant17/1 -> reg_port17/1
  reg_port17/1 -> PortMux_Odd/10
  IP_Constant19/1 -> reg_ip19/1
  reg_ip19/1 -> IPMux_Odd/11
  Port_Constant19/1 -> reg_port19/1
  reg_port19/1 -> PortMux_Odd/11
  IP_Constant21/1 -> reg_ip21/1
  reg_ip21/1 -> IPMux_Odd/12
  Port_Constant21/1 -> reg_port21/1
  reg_port21/1 -> PortMux_Odd/12
  IP_Constant23/1 -> reg_ip23/1
  reg_ip23/1 -> IPMux_Odd/13
  Port_Constant23/1 -> reg_port23/1
  reg_port23/1 -> PortMux_Odd/13
  IP_Constant25/1 -> reg_ip25/1
  reg_ip25/1 -> IPMux_Odd/14
  Port_Constant25/1 -> reg_port25/1
  reg_port25/1 -> PortMux_Odd/14
  IP_Constant27/1 -> reg_ip27/1
  reg_ip27/1 -> IPMux_Odd/15
  Port_Constant27/1 -> reg_port27/1
  reg_port27/1 -> PortMux_Odd/15
  IP_Constant29/1 -> reg_ip29/1
  reg_ip29/1 -> IPMux_Odd/16
  Port_Constant29/1 -> reg_port29/1
  reg_port29/1 -> PortMux_Odd/16
  IP_Constant31/1 -> reg_ip31/1
  reg_ip31/1 -> IPMux_Odd/17
  Port_Constant31/1 -> reg_port31/1
  reg_port31/1 -> PortMux_Odd/17
  IP_Constant2/1 -> reg_ip2/1
  reg_ip2/1 -> IPMux_Even/2
  Port_Constant2/1 -> reg_port2/1
  reg_port2/1 -> PortMux_Even/2
  IP_Constant4/1 -> reg_ip4/1
  reg_ip4/1 -> IPMux_Even/3
  Port_Constant4/1 -> reg_port4/1
  reg_port4/1 -> PortMux_Even/3
  IP_Constant6/1 -> reg_ip6/1
  reg_ip6/1 -> IPMux_Even/4
  Port_Constant6/1 -> reg_port6/1
  reg_port6/1 -> PortMux_Even/4
  IP_Constant8/1 -> reg_ip8/1
  reg_ip8/1 -> IPMux_Even/5
  Port_Constant8/1 -> reg_port8/1
  reg_port8/1 -> PortMux_Even/5
  IP_Constant10/1 -> reg_ip10/1
  reg_ip10/1 -> IPMux_Even/6
  Port_Constant10/1 -> reg_port10/1
  reg_port10/1 -> PortMux_Even/6
  IP_Constant12/1 -> reg_ip12/1
  reg_ip12/1 -> IPMux_Even/7
  Port_Constant12/1 -> reg_port12/1
  reg_port12/1 -> PortMux_Even/7
  IP_Constant14/1 -> reg_ip14/1
  reg_ip14/1 -> IPMux_Even/8
  Port_Constant14/1 -> reg_port14/1
  reg_port14/1 -> PortMux_Even/8
  IP_Constant16/1 -> reg_ip16/1
  reg_ip16/1 -> IPMux_Even/9
  Port_Constant16/1 -> reg_port16/1
  reg_port16/1 -> PortMux_Even/9
  IP_Constant18/1 -> reg_ip18/1
  reg_ip18/1 -> IPMux_Even/10
  Port_Constant18/1 -> reg_port18/1
  reg_port18/1 -> PortMux_Even/10
  IP_Constant20/1 -> reg_ip20/1
  reg_ip20/1 -> IPMux_Even/11
  Port_Constant20/1 -> reg_port20/1
  reg_port20/1 -> PortMux_Even/11
  IP_Constant22/1 -> reg_ip22/1
  reg_ip22/1 -> IPMux_Even/12
  Port_Constant22/1 -> reg_port22/1
  reg_port22/1 -> PortMux_Even/12
  IP_Constant24/1 -> reg_ip24/1
  reg_ip24/1 -> IPMux_Even/13
  Port_Constant24/1 -> reg_port24/1
  reg_port24/1 -> PortMux_Even/13
  IP_Constant26/1 -> reg_ip26/1
  reg_ip26/1 -> IPMux_Even/14
  Port_Constant26/1 -> reg_port26/1
  reg_port26/1 -> PortMux_Even/14
  IP_Constant28/1 -> reg_ip28/1
  reg_ip28/1 -> IPMux_Even/15
  Port_Constant28/1 -> reg_port28/1
  reg_port28/1 -> PortMux_Even/15
  IP_Constant30/1 -> reg_ip30/1
  reg_ip30/1 -> IPMux_Even/16
  Port_Constant30/1 -> reg_port30/1
  reg_port30/1 -> PortMux_Even/16
  IP_Constant32/1 -> reg_ip32/1
  reg_ip32/1 -> IPMux_Even/17
  Port_Constant32/1 -> reg_port32/1
  reg_port32/1 -> PortMux_Even/17
  Num_IPs_Constant/1 -> reg_num_ips/1
  reg_num_ips/1 -> counter_even/3(count_to), counter_odd/3(count_to)
  Gateway Out/1 -> Scope/1
  Gateway Out1/1 -> Scope/2
  Delay_Even/1 -> Logical2/1
  Logical2/1 -> counter_even/1(sync_in)
  Reset_Even/1 -> Logical2/2

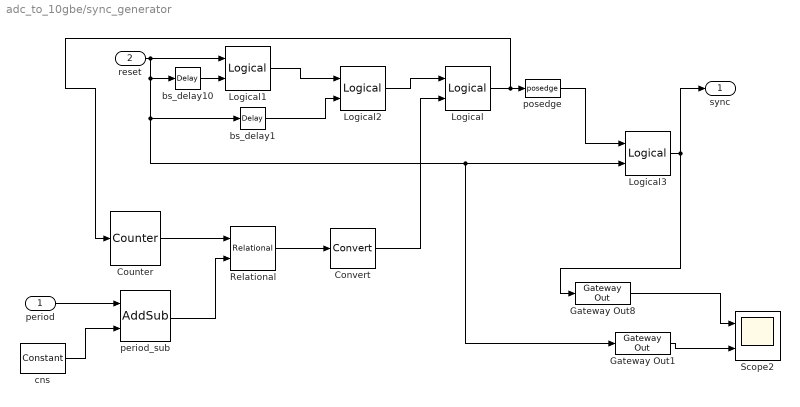
== system adc_to_10gbe/sync_generator ==
  period : Inport  OutDataType=sfix(16)  OutScaling=2^0
  reset : Inport  Port=2  OutDataType=sfix(16)  OutScaling=2^0
  Convert : xbsIndex_r4/Convert  arith_type=Boolean  n_bits=8  bin_pt=6  quantization=Truncate  overflow=Wrap  latency=1  dbl_ovrd=off  pipeline=off  block_type=convert
      settings: xl_area=[0, 0, 0, 0, 0, 0, 0]  block_version=10.1
  Counter : xbsIndex_r4/Counter  cnt_type=Free Running  cnt_to=Inf  operation=Up  start_count=1  cnt_by_val=1  arith_type=Unsigned  n_bits=32  bin_pt=0  load_pin=off  rst=on  en=off  explicit_period=on  period=1  dbl_ovrd=off  use_behavioral_HDL=off  implementation=Fabric  use_rpm=on  block_type=counter
      settings: xl_area=[0, 0, 0, 0, 0, 0, 0]  block_version=10.1
  Gateway Out1 : xbsIndex_r4/Gateway Out  hdl_port=off  timing_constraint=None  locs_specified=off  LOCs={}  block_type=gatewayout
      settings: infoedit="Gateway out block.  Converts Xilinx fixed point inputs into ouputs of type Simulink integer, double, or fixed point.<P><P>Hardware notes:  In hardware these blocks become top level output ports or are discarded, depending on how they are configured."  xl_area=[0, 0, 0, 0, 0, 0, 0]  block_version=10.1
  Gateway Out8 : xbsIndex_r4/Gateway Out  hdl_port=off  timing_constraint=None  locs_specified=off  LOCs={}  block_type=gatewayout
      settings: infoedit="Gateway out block.  Converts Xilinx fixed point inputs into ouputs of type Simulink integer, double, or fixed point.<P><P>Hardware notes:  In hardware these blocks become top level output ports or are discarded, depending on how they are configured."  xl_area=[0, 0, 0, 0, 0, 0, 0]  block_version=10.1
  Logical{,1..3} (4 alike) : xbsIndex_r4/Logical  logical_function=OR  inputs=2  en=off  latency=0  precision=Full  arith_type=Unsigned  n_bits=8  bin_pt=2  align_bp=on  dbl_ovrd=off  block_type=logical
      settings: xl_area=[0, 0, 0, 0, 0, 0, 0]  block_version=10.1
  Relational : xbsIndex_r4/Relational  mode=a>=b  en=off  latency=1  dbl_ovrd=off  block_type=relational
      settings: xl_area=[0, 0, 0, 0, 0, 0, 0]  block_version=10.1
  Scope2 : Scope  NumInputPorts=2
      settings: YMin=-1~-5  YMax=1~5  SaveName=ScopeData6
  bs_delay1 : xbsIndex_r4/Delay  en=off  latency=2  dbl_ovrd=off  reg_retiming=off  block_type=delay
      settings: xl_area=[0, 0, 0, 0, 0, 0, 0]  block_version=10.1
  bs_delay10 : xbsIndex_r4/Delay  en=off  latency=1  dbl_ovrd=off  reg_retiming=off  block_type=delay
      settings: xl_area=[0, 0, 0, 0, 0, 0, 0]  block_version=10.1
  cns : xbsIndex_r4/Constant  arith_type=Unsigned  const=4  n_bits=3  bin_pt=0  explicit_period=off  period=1  equ=P=C  opselect=C  inp2=PCIN>>17  opr=+  inp1=P  carry=CIN  dbl_ovrd=off  block_type=constant
      settings: block_version=10.1
  period_sub : xbsIndex_r4/AddSub  mode=Subtraction  use_carryin=off  use_carryout=off  en=off  latency=0  precision=User Defined  arith_type=Unsigned  n_bits=32  bin_pt=0  quantization=Truncate  overflow=Wrap  dbl_ovrd=off  use_behavioral_HDL=on  hw_selection=Fabric  pipelined=off  use_rpm=on  block_type=addsub
      settings: xl_area=[0, 0, 0, 0, 0, 0, 0]  block_version=10.1
  posedge : casper_library_misc/posedge  Tag=Rising Edge Detector  SystemSampleTime=-1
  sync : Outport  OutDataType=sfix(16)  OutScaling=2^0
  wires:
  Counter/1 -> Relational/1
  Relational/1 -> Convert/1
  Convert/1 -> Logical/2
  Logical/1 -> posedge/1, Counter/1
  reset/1 -> Logical1/1, bs_delay10/1, bs_delay1/1, Logical3/2, Gateway Out1/1
  period/1 -> period_sub/1
  period_sub/1 -> Relational/2
  cns/1 -> period_sub/2
  Gateway Out8/1 -> Scope2/1
  Gateway Out1/1 -> Scope2/2
  bs_delay10/1 -> Logical1/2
  Logical2/1 -> Logical/1
  Logical1/1 -> Logical2/1
  bs_delay1/1 -> Logical2/2
  posedge/1 -> Logical3/1
  Logical3/1 -> sync/1, Gateway Out8/1

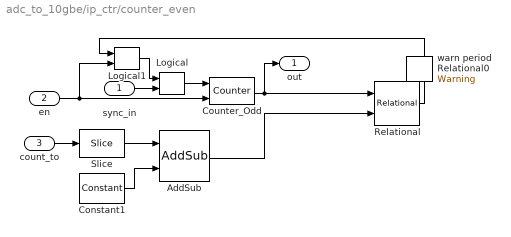
== system adc_to_10gbe/ip_ctr/counter_even ==
  sync_in : Inport  OutDataType=sfix(16)  OutScaling=2^0
  en : Inport  Port=2  OutDataType=sfix(16)  OutScaling=2^0
  count_to : Inport  Port=3  OutDataType=sfix(16)  OutScaling=2^0
  AddSub : xbsIndex_r4/AddSub  mode=Subtraction  use_carryin=off  use_carryout=off  en=off  latency=0  precision=Full  arith_type=Unsigned  n_bits=8  bin_pt=2  quantization=Truncate  overflow=Wrap  dbl_ovrd=off  use_behavioral_HDL=on  hw_selection=Fabric  pipelined=off  use_rpm=on  block_type=addsub
      settings: xl_area=[0, 0, 0, 0, 0, 0, 0]  block_version=10.1
  Constant1 : xbsIndex_r4/Constant  arith_type=Unsigned  const=1  n_bits=4  bin_pt=0  explicit_period=on  period=1  equ=P=C  opselect=C  inp2=PCIN>>17  opr=+  inp1=P  carry=CIN  dbl_ovrd=off  block_type=constant
      settings: block_version=10.1
  Counter_Odd : xbsIndex_r4/Counter  cnt_type=Free Running  cnt_to=Inf  operation=Up  start_count=0  cnt_by_val=1  arith_type=Unsigned  n_bits=4  bin_pt=0  load_pin=off  rst=on  en=on  explicit_period=off  period=1  dbl_ovrd=off  use_behavioral_HDL=off  implementation=Fabric  use_rpm=on  block_type=counter
      settings: xl_area=[0, 0, 0, 0, 0, 0, 0]  block_version=10.1
  Logical : xbsIndex_r4/Logical  logical_function=OR  inputs=2  en=off  latency=0  precision=Full  arith_type=Unsigned  n_bits=8  bin_pt=2  align_bp=on  dbl_ovrd=off  block_type=logical
      settings: xl_area=[0, 0, 0, 0, 0, 0, 0]  block_version=10.1
  Logical1 : xbsIndex_r4/Logical  logical_function=AND  inputs=2  en=off  latency=0  precision=Full  arith_type=Unsigned  n_bits=8  bin_pt=2  align_bp=on  dbl_ovrd=off  block_type=logical
      settings: xl_area=[0, 0, 0, 0, 0, 0, 0]  block_version=10.1
  Relational : xbsIndex_r4/Relational  mode=a=b  en=off  latency=1  dbl_ovrd=off  block_type=relational
      settings: xl_area=[0, 0, 0, 0, 0, 0, 0]  block_version=10.1
  Slice : xbsIndex_r4/Slice  nbits=4  boolean_output=off  mode=Lower Bit Location + Width  bit1=0  base1=MSB of Input  bit0=1  base0=LSB of Input  dbl_ovrd=off  block_type=slice
      settings: infoedit="Extracts a given range of bits from each input sample and presents it at the output.  The output type is ordinarily unsigned with binary point at zero, but can be Boolean when the slice is one bit wide.<P><P>Hardware notes: In hardware this block costs nothing."  block_version=10.1
  warn period Relational0 : xbsReplacements_r4/Warning  SystemSampleTime=-1  period=1
  out : Outport  OutDataType=sfix(16)  OutScaling=2^0
  wires:
  en/1 -> Logical1/2, Counter_Odd/2
  Counter_Odd/1 -> Relational/1, out/1
  Logical/1 -> Counter_Odd/1
  Relational/1 -> Logical1/1
  Logical1/1 -> Logical/1
  Slice/1 -> AddSub/1
  AddSub/1 -> Relational/2
  Constant1/1 -> AddSub/2
  sync_in/1 -> Logical/2
  count_to/1 -> Slice/1

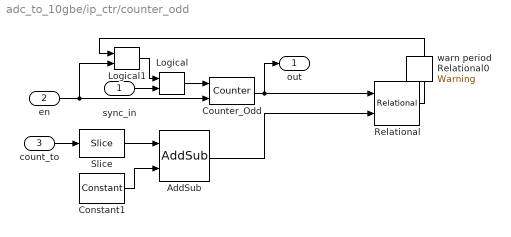
== system adc_to_10gbe/ip_ctr/counter_odd ==
  sync_in : Inport  OutDataType=sfix(16)  OutScaling=2^0
  en : Inport  Port=2  OutDataType=sfix(16)  OutScaling=2^0
  count_to : Inport  Port=3  OutDataType=sfix(16)  OutScaling=2^0
  AddSub : xbsIndex_r4/AddSub  mode=Subtraction  use_carryin=off  use_carryout=off  en=off  latency=0  precision=Full  arith_type=Unsigned  n_bits=8  bin_pt=2  quantization=Truncate  overflow=Wrap  dbl_ovrd=off  use_behavioral_HDL=on  hw_selection=Fabric  pipelined=off  use_rpm=on  block_type=addsub
      settings: xl_area=[0, 0, 0, 0, 0, 0, 0]  block_version=10.1
  Constant1 : xbsIndex_r4/Constant  arith_type=Unsigned  const=1  n_bits=4  bin_pt=0  explicit_period=on  period=1  equ=P=C  opselect=C  inp2=PCIN>>17  opr=+  inp1=P  carry=CIN  dbl_ovrd=off  block_type=constant
      settings: block_version=10.1
  Counter_Odd : xbsIndex_r4/Counter  cnt_type=Free Running  cnt_to=Inf  operation=Up  start_count=0  cnt_by_val=1  arith_type=Unsigned  n_bits=4  bin_pt=0  load_pin=off  rst=on  en=on  explicit_period=off  period=1  dbl_ovrd=off  use_behavioral_HDL=off  implementation=Fabric  use_rpm=on  block_type=counter
      settings: xl_area=[0, 0, 0, 0, 0, 0, 0]  block_version=10.1
  Logical : xbsIndex_r4/Logical  logical_function=OR  inputs=2  en=off  latency=0  precision=Full  arith_type=Unsigned  n_bits=8  bin_pt=2  align_bp=on  dbl_ovrd=off  block_type=logical
      settings: xl_area=[0, 0, 0, 0, 0, 0, 0]  block_version=10.1
  Logical1 : xbsIndex_r4/Logical  logical_function=AND  inputs=2  en=off  latency=0  precision=Full  arith_type=Unsigned  n_bits=8  bin_pt=2  align_bp=on  dbl_ovrd=off  block_type=logical
      settings: xl_area=[0, 0, 0, 0, 0, 0, 0]  block_version=10.1
  Relational : xbsIndex_r4/Relational  mode=a=b  en=off  latency=1  dbl_ovrd=off  block_type=relational
      settings: xl_area=[0, 0, 0, 0, 0, 0, 0]  block_version=10.1
  Slice : xbsIndex_r4/Slice  nbits=4  boolean_output=off  mode=Lower Bit Location + Width  bit1=0  base1=MSB of Input  bit0=1  base0=LSB of Input  dbl_ovrd=off  block_type=slice
      settings: infoedit="Extracts a given range of bits from each input sample and presents it at the output.  The output type is ordinarily unsigned with binary point at zero, but can be Boolean when the slice is one bit wide.<P><P>Hardware notes: In hardware this block costs nothing."  block_version=10.1
  warn period Relational0 : xbsReplacements_r4/Warning  SystemSampleTime=-1  period=1
  out : Outport  OutDataType=sfix(16)  OutScaling=2^0
  wires:
  en/1 -> Logical1/2, Counter_Odd/2
  Counter_Odd/1 -> Relational/1, out/1
  Logical/1 -> Counter_Odd/1
  Relational/1 -> Logical1/1
  Logical1/1 -> Logical/1
  Slice/1 -> AddSub/1
  AddSub/1 -> Relational/2
  Constant1/1 -> AddSub/2
  sync_in/1 -> Logical/2
  count_to/1 -> Slice/1
